simulink model "p_isled_zap"  (R2017b)
settings: Solver=VariableStepAuto  StartTime=0.0  StopTime=t_final  MaxStep=0.001  RelTol=1e-3
undefined symbols (not defined in the file): K1, K2, Kp, Kpa, T0, T1
settings Model: Creator=Anton Mayorov  LastModifiedBy=bedla

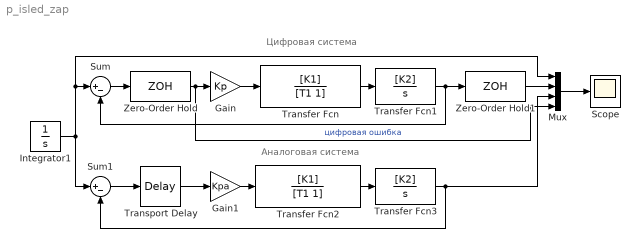
== system p_isled_zap ==
  note: Аналоговая система
  note: Цифровая система
  Gain : Gain  Gain=Kp
  Gain1 : Gain  Gain=Kpa
  Integrator1 : Integrator  InitialCondition=1
  Mux : Mux
  Scope : Scope
  Sum : Sum  Inputs=|+-
  Sum1 : Sum  Inputs=|+-
  Transfer Fcn : TransferFcn  Numerator=[K1]  Denominator=[T1 1]
  Transfer Fcn1 : TransferFcn  Numerator=[K2]  Denominator=[1 0]
  Transfer Fcn2 : TransferFcn  Numerator=[K1]  Denominator=[T1 1]
  Transfer Fcn3 : TransferFcn  Numerator=[K2]  Denominator=[1 0]
  Transport Delay : TransportDelay  DelayTime=0.5*T0
  Zero-Order Hold : ZeroOrderHold  SampleTime=T0
  Zero-Order Hold1 : ZeroOrderHold  SampleTime=T0
  wires:
  Zero-Order Hold/1 -> Mux/4, Gain/1  "цифровая ошибка"
  Transfer Fcn/1 -> Transfer Fcn1/1
  Mux/1 -> Scope/1
  Gain/1 -> Transfer Fcn/1
  Transfer Fcn1/1 -> Sum/2, Zero-Order Hold1/1
  Sum/1 -> Zero-Order Hold/1
  Integrator1/1 -> Mux/1, Sum/1, Sum1/1
  Sum1/1 -> Transport Delay/1
  Transfer Fcn3/1 -> Mux/3, Sum1/2
  Gain1/1 -> Transfer Fcn2/1
  Transfer Fcn2/1 -> Transfer Fcn3/1
  Zero-Order Hold1/1 -> Mux/2
  Transport Delay/1 -> Gain1/1
